simulink model "gabelstapler_Simulink_ungeregelt"  (R2025a)
settings: Solver=VariableStepAuto  StartTime=0.0  StopTime=100  RelTol=1e-3
undefined symbols (not defined in the file): d, d_gtr, i_Getriebe, k, k_Acc, k_D, k_e, k_I, k_Motor, k_P, L_Motor, m_g, R_Motor, r_R, theta_s
libraries: simulink x12
settings Model: Creator=Manuel  LastModifiedBy=gerke

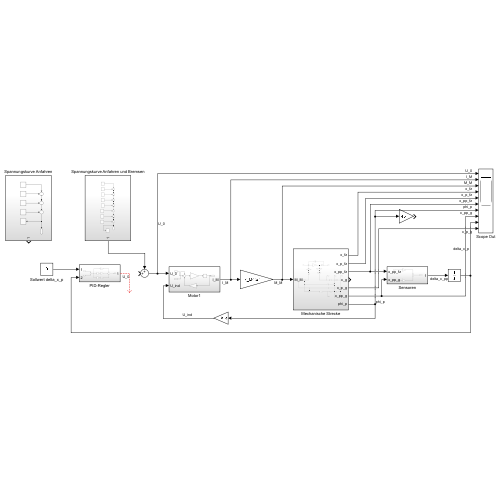
[thumbnail: Simulink's stored preview of the top-level diagram]
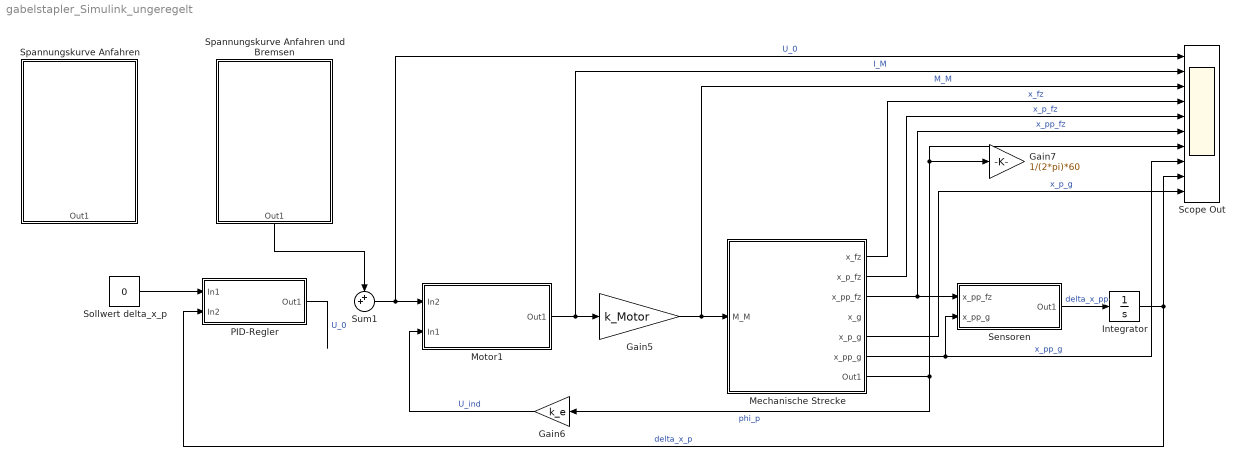
== system gabelstapler_Simulink_ungeregelt ==
  Gain5 : Gain  Gain=k_Motor
  Gain6 : Gain  Gain=k_e
  Gain7 : Gain  Gain=1/(2*pi)*60
  Integrator : Integrator
  Mechanische Strecke : Subsystem
  Motor1 : Subsystem
  PID-Regler : Subsystem
  Scope Out : Scope  NumInputPorts=10
      settings: ActiveDisplayYMinimum=-37.500000000000064  ActiveDisplayYMaximum=37.500000000000014  DataLoggingVariableName=Scope_out
  Sensoren : Subsystem
  Sollwert delta_x_p : Constant  Value=0
  Spannungskurve Anfahren : Subsystem
  Spannungskurve Anfahren und Bremsen : Subsystem
  Sum1 : Sum  Inputs=++|
  wires:
  PID-Regler/1(Out1) -> ?  "U_0"
  Mechanische Strecke/6(x_pp_g) -> Sensoren/2(x_pp_g), Scope Out/8  "x_pp_g"
  Mechanische Strecke/3(x_pp_fz) -> Sensoren/1(x_pp_fz), Scope Out/6  "x_pp_fz"
  Motor1/1(Out1) -> Scope Out/2, Gain5/1  "I_M"
  Sum1/1 -> Motor1/1(In2), Scope Out/1  "U_0"
  Gain5/1 -> Mechanische Strecke/1(M_M), Scope Out/3  "M_M"
  Mechanische Strecke/7(Out1) -> Scope Out/7, Gain7/1, Gain6/1  "phi_p"
  Gain6/1 -> Motor1/2(In1)  "U_ind"
  Mechanische Strecke/2(x_p_fz) -> Scope Out/5  "x_p_fz"
  Mechanische Strecke/1(x_fz) -> Scope Out/4  "x_fz"
  Sollwert delta_x_p/1 -> PID-Regler/1(In1)
  Sensoren/1(Out1) -> Integrator/1  "delta_x_pp"
  Integrator/1 -> Scope Out/9, PID-Regler/2(In2)  "delta_x_p"
  Spannungskurve Anfahren und Bremsen/1(Out1) -> Sum1/1
  Mechanische Strecke/5(x_p_g) -> Scope Out/10  "x_p_g"

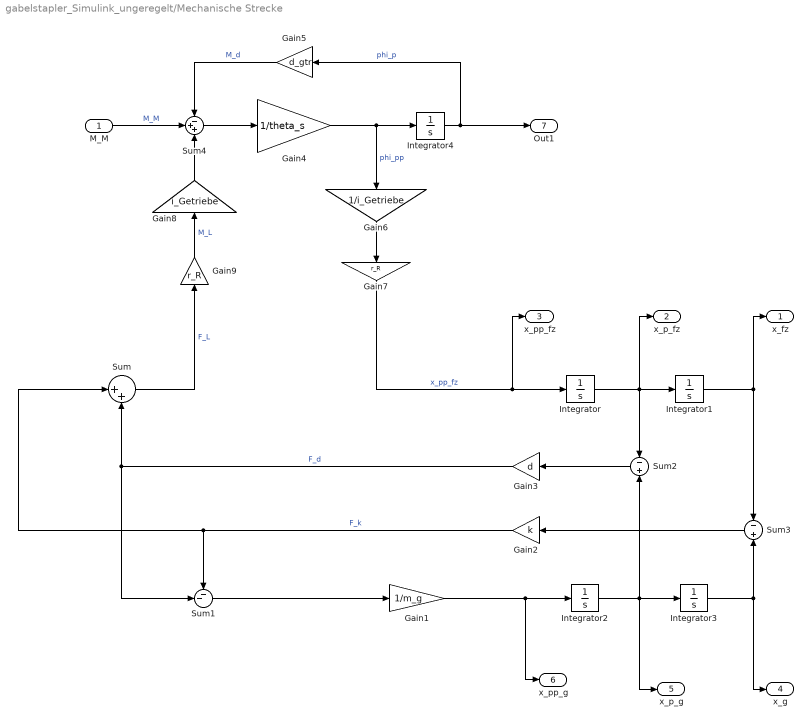
== system gabelstapler_Simulink_ungeregelt/Mechanische Strecke ==
  M_M : Inport
  Gain1 : Gain  Gain=1/m_g
  Gain2 : Gain  Gain=k
  Gain3 : Gain  Gain=d
  Gain4 : Gain  Gain=1/theta_s
  Gain5 : Gain  Gain=d_gtr
  Gain6 : Gain  Gain=1/i_Getriebe
  Gain7 : Gain  Gain=r_R
  Gain8 : Gain  Gain=i_Getriebe
  Gain9 : Gain  Gain=r_R
  Integrator{,1..4} (5 alike) : Integrator
  Sum : Sum  Inputs=|++
  Sum1 : Sum  Inputs=--|
  Sum2 : Sum  Inputs=-|+
  Sum3 : Sum  Inputs=-|+
  Sum4 : Sum  Inputs=-++
  x_fz : Outport
  x_p_fz : Outport  Port=2
  x_pp_fz : Outport  Port=3
  x_g : Outport  Port=4
  x_p_g : Outport  Port=5
  x_pp_g : Outport  Port=6
  Out1 : Outport  Port=7
  wires:
  Integrator/1 -> Sum2/1, Integrator1/1, x_p_fz/1
  Integrator1/1 -> Sum3/1, x_fz/1
  Integrator2/1 -> x_p_g/1, Integrator3/1, Sum2/2
  Integrator3/1 -> x_g/1, Sum3/2
  Sum1/1 -> Gain1/1
  Gain1/1 -> x_pp_g/1, Integrator2/1
  Sum3/1 -> Gain2/1
  Sum2/1 -> Gain3/1
  Gain3/1 -> Sum1/2, Sum/2  "F_d"
  Gain2/1 -> Sum/1, Sum1/1  "F_k"
  Gain5/1 -> Sum4/1  "M_d"
  Gain4/1 -> Integrator4/1, Gain6/1  "phi_pp"
  Sum/1 -> Gain9/1  "F_L"
  Gain8/1 -> Sum4/3
  M_M/1 -> Sum4/2  "M_M"
  Gain9/1 -> Gain8/1  "M_L"
  Integrator4/1 -> Gain5/1, Out1/1  "phi_p"
  Gain6/1 -> Gain7/1
  Sum4/1 -> Gain4/1
  Gain7/1 -> x_pp_fz/1, Integrator/1  "x_pp_fz"

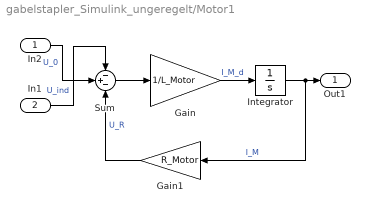
== system gabelstapler_Simulink_ungeregelt/Motor1 ==
  In2 : Inport
  In1 : Inport  Port=2
  Gain : Gain  Gain=1/L_Motor
  Gain1 : Gain  Gain=R_Motor
  Integrator : Integrator
  Sum : Sum  Inputs=-+-
  Out1 : Outport
  wires:
  Gain1/1 -> Sum/3  "U_R"
  Sum/1 -> Gain/1
  In2/1 -> Sum/2  "U_0"
  In1/1 -> Sum/1  "U_ind"
  Integrator/1 -> Gain1/1, Out1/1  "I_M"
  Gain/1 -> Integrator/1  "I_M_d"

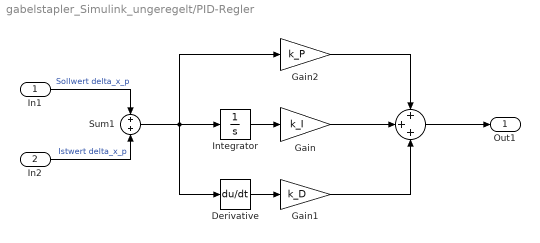
== system gabelstapler_Simulink_ungeregelt/PID-Regler ==
  In1 : Inport
  In2 : Inport  Port=2
  " " : Sum  Inputs=+++
  Derivative : Derivative
  Gain : Gain  Gain=k_I
  Gain1 : Gain  Gain=k_D
  Gain2 : Gain  Gain=k_P
  Integrator : Integrator
  Sum1 : Sum  Inputs=+|+
  Out1 : Outport
  wires:
  Integrator/1 -> Gain/1
  Gain/1 -> " "/2
  " "/1 -> Out1/1
  Derivative/1 -> Gain1/1
  Gain1/1 -> " "/3
  Gain2/1 -> " "/1
  In2/1 -> Sum1/2  "Istwert delta_x_p"
  In1/1 -> Sum1/1  "Sollwert delta_x_p"
  Sum1/1 -> Integrator/1, Derivative/1, Gain2/1

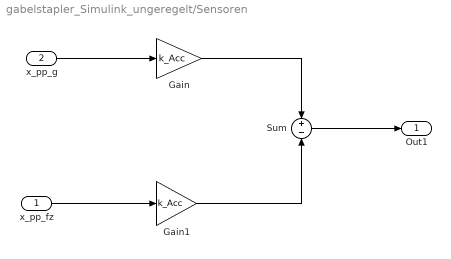
== system gabelstapler_Simulink_ungeregelt/Sensoren ==
  x_pp_fz : Inport
  x_pp_g : Inport  Port=2
  Gain : Gain  Gain=k_Acc
  Gain1 : Gain  Gain=k_Acc
  Sum : Sum  Inputs=+|-
  Out1 : Outport
  wires:
  x_pp_g/1 -> Gain/1
  x_pp_fz/1 -> Gain1/1
  Gain/1 -> Sum/1
  Gain1/1 -> Sum/2
  Sum/1 -> Out1/1

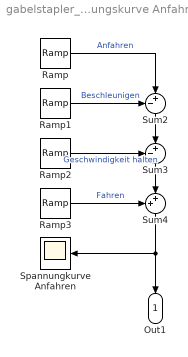
== system gabelstapler_Simulink_ungeregelt/Spannungskurve Anfahren ==
  Ramp : simulink/Sources/Ramp  slope=15  start=10  InitialOutput=0
  Ramp1 : simulink/Sources/Ramp  slope=15  start=12  InitialOutput=0
  Ramp2 : simulink/Sources/Ramp  slope=7.5  start=15  InitialOutput=0
  Ramp3 : simulink/Sources/Ramp  slope=7.5  start=17  InitialOutput=0
  Spannungkurve Anfahren : Scope
      settings: ActiveDisplayYMinimum=-5.6213254343023973  ActiveDisplayYMaximum=35.7224245656976  DataLoggingVariableName=ScopeData2
  Sum2 : Sum  Inputs=-+|
  Sum3 : Sum  Inputs=-+|
  Sum4 : Sum  Inputs=++|
  Out1 : Outport
  wires:
  Ramp3/1 -> Sum4/1  "Fahren"
  Ramp/1 -> Sum2/2  "Anfahren"
  Sum3/1 -> Sum4/2
  Sum2/1 -> Sum3/2
  Ramp2/1 -> Sum3/1  "Geschwindigkeit halten"
  Ramp1/1 -> Sum2/1  "Beschleunigen"
  Sum4/1 -> Out1/1, Spannungkurve Anfahren/1

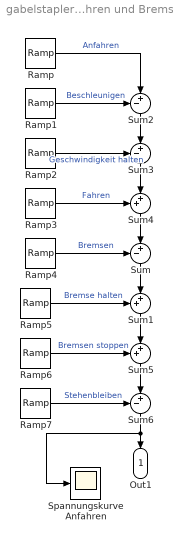
== system gabelstapler_Simulink_ungeregelt/Spannungskurve Anfahren und Bremsen ==
  Ramp : simulink/Sources/Ramp  slope=15  start=10  InitialOutput=0
  Ramp1 : simulink/Sources/Ramp  slope=15  start=12  InitialOutput=0
  Ramp2 : simulink/Sources/Ramp  slope=7.5  start=15  InitialOutput=0
  Ramp3 : simulink/Sources/Ramp  slope=7.5  start=17  InitialOutput=0
  Ramp4 : simulink/Sources/Ramp  slope=15  start=40  InitialOutput=0
  Ramp5 : simulink/Sources/Ramp  slope=15  start=43  InitialOutput=0
  Ramp6 : simulink/Sources/Ramp  slope=15  start=49  InitialOutput=0
  Ramp7 : simulink/Sources/Ramp  slope=15  start=51  InitialOutput=0
  Spannungskurve Anfahren : Scope
      settings: ActiveDisplayYMinimum=-37.500000000000064  ActiveDisplayYMaximum=37.500000000000014  DataLoggingVariableName=ScopeData3
  Sum{,2..3,6} (4 alike) : Sum  Inputs=-+|
  Sum1 : Sum  Inputs=++|
  Sum4 : Sum  Inputs=++|
  Sum5 : Sum  Inputs=++|
  Out1 : Outport
  wires:
  Ramp3/1 -> Sum4/1  "Fahren"
  Ramp/1 -> Sum2/2  "Anfahren"
  Sum3/1 -> Sum4/2
  Sum2/1 -> Sum3/2
  Ramp2/1 -> Sum3/1  "Geschwindigkeit halten"
  Ramp1/1 -> Sum2/1  "Beschleunigen"
  Ramp4/1 -> Sum/1  "Bremsen"
  Sum4/1 -> Sum/2
  Ramp5/1 -> Sum1/1  "Bremse halten"
  Sum/1 -> Sum1/2
  Ramp6/1 -> Sum5/1  "Bremsen stoppen"
  Sum1/1 -> Sum5/2
  Sum5/1 -> Sum6/2
  Ramp7/1 -> Sum6/1  "Stehenbleiben"
  Sum6/1 -> Spannungskurve Anfahren/1, Out1/1
